simulink model "open_loop"  (R2016b)
settings: Solver=FixedStepAuto  StartTime=0.0  StopTime=10.0  FixedStep=1/100  RelTol=1e-3  AbsTol=1e-3
model workspace: external: MATLAB File /home/frehage/ownCloud/TEACHING/Embeded Control Systems - SSY190/2017/StudentRepo/crazyflie-firmware/simulink-model/params.m (data not in the file)
undefined symbols (not defined in the file or in its folder): b, g, k, m
libraries: nesl_utility x7
settings Model: Creator=Jocke  LastModifiedBy=frehage
settings SimscapeCC: SimscapeLogType=all  SimscapeLogDataHistory=10000

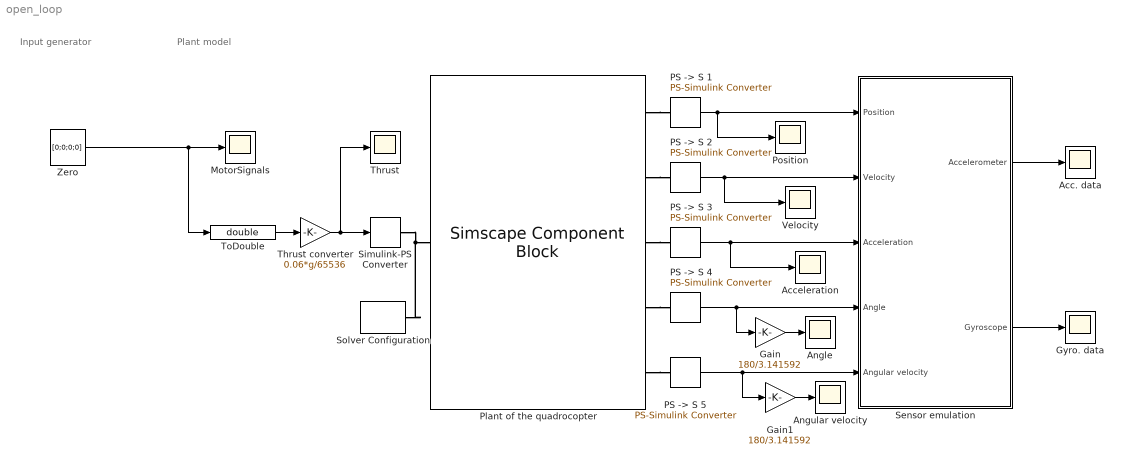
== system open_loop ==
  note: Plant model
  note: Input generator
  Acc. data : Scope
  Acceleration : Scope
  Angle : Scope
  Angular velocity : Scope
  Gain : Gain  Gain=180/3.141592
  Gain1 : Gain  Gain=180/3.141592
  Gyro. data : Scope
  MotorSignals : Scope
  PS -> S {1..5} (5 alike) : nesl_utility/PS-Simulink Converter  PhysicalDomain=network_engine_domain  SubClassName=ps_output  LeftPortType=input  RightPortType=output  PseudoPeriodic=off  Frequencies=[]  Unit=1  AffineConversion=off
  Plant of the quadrocopter : SimscapeComponentBlock  SourceFile=plant  ComponentPath=plant  ComponentVariants=plant  ComponentVariantNames=plant  ClassName=plant  SchemaVersion=1  m=m kg  g=g m/s^2  d=d m  k=b  b=k
      settings: CopyFcn=simscape.engine.sli.internal.componentblockcallback(gcbh,'COPY')  PreCopyFcn=simscape.engine.sli.internal.componentblockcallback(gcbh,'PRECOPY')  PreDeleteFcn=simscape.engine.sli.internal.componentblockcallback(gcbh,'PREDELETE')
      mask Type: Plant of quadrocopter
      mask Display:
      | disp('Simscape\n\n\n')
      | disp('\n\n\nplant');
      | color('red');
      | port_label('RConn', 5,'Angular velocity');
      | port_label('RConn', 4,'Angle');
      | port_label('RConn', 3,'Acceleration');
      | port_label('RConn', 2,'Velocity');
      | port_label('RConn', 1,'Position');
      | port_label('LConn', 1,'Thrust');
  Position : Scope
  Sensor emulation : Subsystem
  Simulink-PS Converter : nesl_utility/Simulink-PS Converter  PhysicalDomain=network_engine_domain  SubClassName=ps_input  LeftPortType=input  RightPortType=output  PseudoPeriodic=off  Frequencies=[]  NoiseDistribution=none  NoiseParameters=[]  Unit=1  AffineConversion=off  InputFiltering=off  SimscapeFilterOrder=1  InputFilterTimeConstant=0.001  UdotUserProvided=1
  Solver Configuration : nesl_utility/Solver Configuration  PhysicalDomain=network_engine_domain  SubClassName=solver  LeftPortType=input  RightPortType=generic  Accelerate=off  Tones=[]  Harmonics=[]  SimulateNoise=off  Profile=off  UseLocalSampling=off  EnableSwitchedLinearOptims=on  FrequencyDomain=off  UseCCode=off  RelTol=0.001  AbsTol=1e-06  MinStep=1e-09  ToWorkspace=off  RevertToSquareIcSolve=off  NumHomotopyIterations=100  PhasorMode=off  PhasorModeNumHarmonics=1  OverrideAbsTol=off  DoDC=off  ResidualTolerance=1e-09  UseLocalSolver=off  LocalSolverChoice=NE_BACKWARD_EULER_ADVANCER  LocalSolverSampleTime=0.001  DoFixedCost=off  MaxNonlinIter=3  MaxModeIter=2  LinearAlgebra=Sparse  DelaysMemoryBudget=1024  AutomaticFiltering=on  FilteringTimeConstant=0.001
  Thrust : Scope
  Thrust converter : Gain  Gain=0.06*g/65536
  ToDouble : DataTypeConversion  OutDataTypeStr=double  RndMeth=Round  SaturateOnIntegerOverflow=on
  Velocity : Scope
  Zero : Constant  Value=[0;0;0;0]  VectorParams1D=off  OutDataTypeStr=uint16
  wires:
  "PS -> S 5"/1 -> Gain1/1, Sensor emulation/5(Angular velocity)
  "PS -> S 4"/1 -> Gain/1, Sensor emulation/4(Angle)
  "PS -> S 3"/1 -> Sensor emulation/3(Acceleration), Acceleration/1
  "PS -> S 2"/1 -> Sensor emulation/2(Velocity), Velocity/1
  Sensor emulation/2(Gyroscope) -> Gyro. data/1
  Sensor emulation/1(Accelerometer) -> Acc. data/1
  Zero/1 -> MotorSignals/1, ToDouble/1
  "PS -> S 1"/1 -> Position/1, Sensor emulation/1(Position)
  Gain/1 -> Angle/1
  Gain1/1 -> Angular velocity/1
  ToDouble/1 -> Thrust converter/1
  Thrust converter/1 -> Thrust/1, Simulink-PS Converter/1
  connections:
  Plant of the quadrocopter/LConn1 -- Simulink-PS Converter/RConn1 -- Solver Configuration/RConn1
  Plant of the quadrocopter/RConn2 -- "PS -> S 2"/LConn1
  Plant of the quadrocopter/RConn1 -- "PS -> S 1"/LConn1
  Plant of the quadrocopter/RConn4 -- "PS -> S 4"/LConn1
  Plant of the quadrocopter/RConn5 -- "PS -> S 5"/LConn1
  Plant of the quadrocopter/RConn3 -- "PS -> S 3"/LConn1

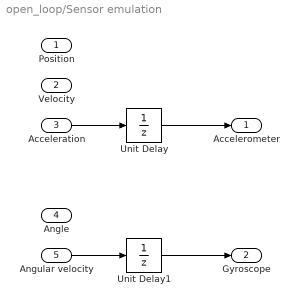
== system open_loop/Sensor emulation ==
  Position : Inport  OutDataTypeStr=double  PortDimensions=3
  Velocity : Inport  Port=2  OutDataTypeStr=double  PortDimensions=3
  Acceleration : Inport  Port=3  OutDataTypeStr=double  PortDimensions=3
  Angle : Inport  Port=4  OutDataTypeStr=double  PortDimensions=3
  Angular velocity : Inport  Port=5  OutDataTypeStr=double  PortDimensions=3
  Unit Delay : UnitDelay  SampleTime=-1
  Unit Delay1 : UnitDelay  SampleTime=-1
  Accelerometer : Outport
  Gyroscope : Outport  Port=2
  wires:
  Acceleration/1 -> Unit Delay/1
  Unit Delay/1 -> Accelerometer/1
  Angular velocity/1 -> Unit Delay1/1
  Unit Delay1/1 -> Gyroscope/1
